simulink model "LONGITUDINAL_VEHICL_DYNAMICS_Model"  (R2024b)
settings: Solver=VariableStepAuto  StartTime=0.0  StopTime=10.0  RelTol=1e-3
values from neighbouring files (symbols this model uses):
  acceleration_due_to_gravity_cst = 9.81    [LONGITUDINAL_VEHICL_DYNAMICS_Constant.m]
  C_rr = 0.010    (= 0.01)    [LONGITUDINAL_VEHICL_DYNAMICS_Constant.m]
  k_drag = 0.40    (= 0.4)    [LONGITUDINAL_VEHICL_DYNAMICS_Constant.m]
  mass_of_the_vehicle = 1500    [LONGITUDINAL_VEHICL_DYNAMICS_Constant.m]
  max_drive_wheel_torque_cst = 2200    [LONGITUDINAL_VEHICL_DYNAMICS_Constant.m]
  maxi_brake_torque_per_wheel_cst = 1500    [LONGITUDINAL_VEHICL_DYNAMICS_Constant.m]
  Wheel_Radius_cst = 0.30    (= 0.3)    [LONGITUDINAL_VEHICL_DYNAMICS_Constant.m]
settings Model: Creator=LENOVO  LastModifiedBy=LENOVO

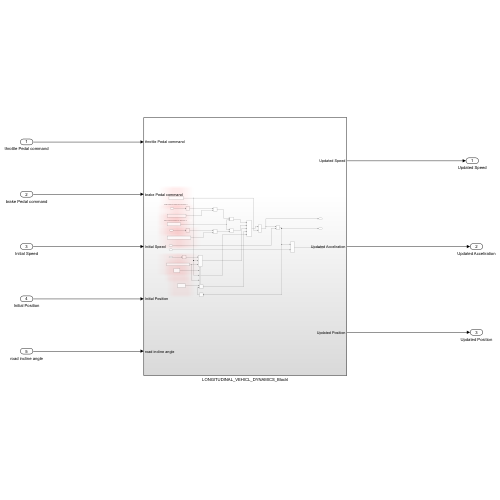
[thumbnail: Simulink's stored preview of the top-level diagram]
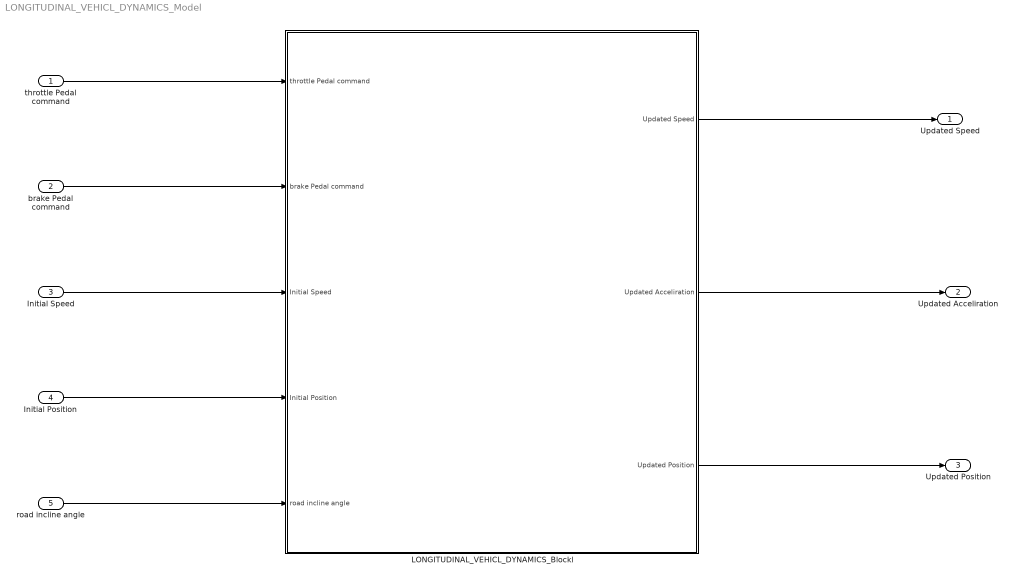
== system LONGITUDINAL_VEHICL_DYNAMICS_Model ==
  throttle Pedal command : Inport  OutMin=0  OutMax=1  OutDataTypeStr=double
  brake Pedal command : Inport  Port=2  OutMin=0  OutMax=1  OutDataTypeStr=double
  Initial Speed : Inport  Port=3
  Initial Position : Inport  Port=4
  road incline angle : Inport  Port=5
  LONGITUDINAL_VEHICL_DYNAMICS_Blockl : Subsystem
  Updated Speed : Outport
  Updated Acceliration : Outport  Port=2
  Updated Position : Outport  Port=3
  wires:
  throttle Pedal command/1 -> LONGITUDINAL_VEHICL_DYNAMICS_Blockl/1(throttle Pedal command)
  brake Pedal command/1 -> LONGITUDINAL_VEHICL_DYNAMICS_Blockl/2(brake Pedal command)
  Initial Speed/1 -> LONGITUDINAL_VEHICL_DYNAMICS_Blockl/3(Initial Speed)
  Initial Position/1 -> LONGITUDINAL_VEHICL_DYNAMICS_Blockl/4(Initial Position)
  road incline angle/1 -> LONGITUDINAL_VEHICL_DYNAMICS_Blockl/5(road incline angle)
  LONGITUDINAL_VEHICL_DYNAMICS_Blockl/1(Updated Speed) -> Updated Speed/1
  LONGITUDINAL_VEHICL_DYNAMICS_Blockl/2(Updated Acceliration) -> Updated Acceliration/1
  LONGITUDINAL_VEHICL_DYNAMICS_Blockl/3(Updated Position) -> Updated Position/1

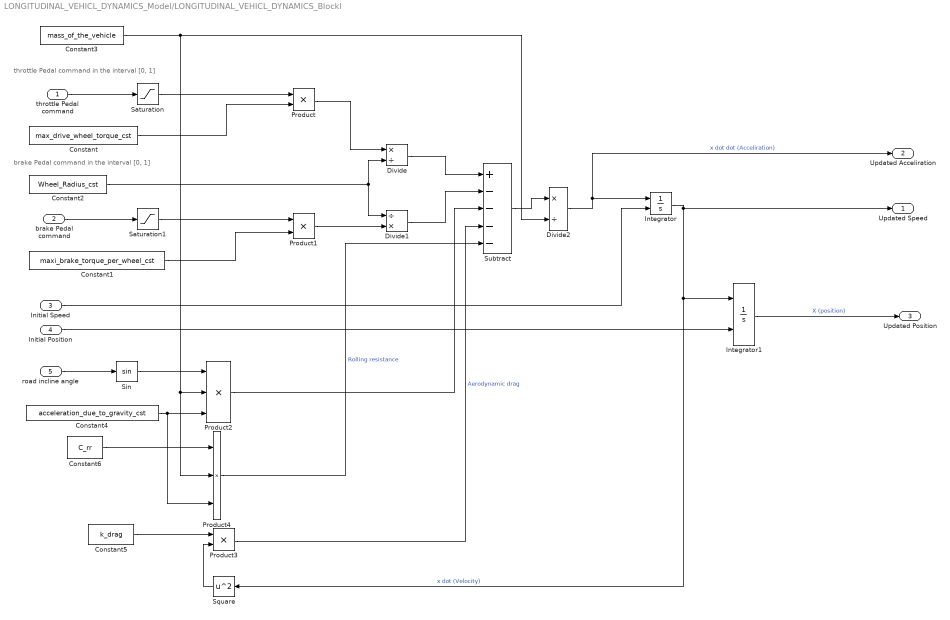
== system LONGITUDINAL_VEHICL_DYNAMICS_Model/LONGITUDINAL_VEHICL_DYNAMICS_Blockl ==
  note: throttle Pedal command in the interval [0, 1]
  note: brake Pedal command in the interval [0, 1]
  throttle Pedal command : Inport  OutMin=0  OutMax=1  OutDataTypeStr=double
  brake Pedal command : Inport  Port=2  OutMin=0  OutMax=1  OutDataTypeStr=double
  Initial Speed : Inport  Port=3
  Initial Position : Inport  Port=4
  road incline angle : Inport  Port=5
  Constant : Constant  Value=max_drive_wheel_torque_cst
  Constant1 : Constant  Value=maxi_brake_torque_per_wheel_cst
  Constant2 : Constant  Value=Wheel_Radius_cst
  Constant3 : Constant  Value=mass_of_the_vehicle
  Constant4 : Constant  Value=acceleration_due_to_gravity_cst
  Constant5 : Constant  Value=k_drag
  Constant6 : Constant  Value=C_rr
  Divide : Product  Inputs=*/
  Divide1 : Product  Inputs=/*
  Divide2 : Product  Inputs=*/
  Integrator : Integrator  InitialConditionSource=external
  Integrator1 : Integrator  InitialConditionSource=external
  Product : Product
  Product1 : Product
  Product2 : Product  Inputs=3
  Product3 : Product
  Product4 : Product  Inputs=3
  Saturation : Saturate
  Saturation1 : Saturate
  Sin : Trigonometry
  Square : Math  Operator=square
  Subtract : Sum  Inputs=+----
  Updated Speed : Outport
  Updated Acceliration : Outport  Port=2
  Updated Position : Outport  Port=3
  wires:
  Subtract/1 -> Divide2/1
  Constant6/1 -> Product4/1
  Constant4/1 -> Product4/3, Product2/3
  Initial Position/1 -> Integrator1/2
  Divide2/1 -> Updated Acceliration/1, Integrator/1  "x dot dot (Acceliration)"
  Saturation/1 -> Product/1
  Integrator/1 -> Updated Speed/1, Integrator1/1, Square/1  "x dot (Velocity)"
  Constant2/1 -> Divide1/1, Divide/2
  Product3/1 -> Subtract/4  "Aerodynamic drag"
  Saturation1/1 -> Product1/1
  Constant3/1 -> Divide2/2, Product4/2, Product2/2
  Product2/1 -> Subtract/3
  brake Pedal command/1 -> Saturation1/1
  Constant5/1 -> Product3/1
  Square/1 -> Product3/2
  Divide1/1 -> Subtract/2
  Initial Speed/1 -> Integrator/2
  Product4/1 -> Subtract/5  "Rolling resistance"
  Constant/1 -> Product/2
  Divide/1 -> Subtract/1
  Sin/1 -> Product2/1
  Integrator1/1 -> Updated Position/1  "X (position)"
  Constant1/1 -> Product1/2
  Product1/1 -> Divide1/2
  throttle Pedal command/1 -> Saturation/1
  road incline angle/1 -> Sin/1
  Product/1 -> Divide/1
